simulink model "Temperature_Controller"  (R2024b)
settings: Solver=VariableStepAuto  StartTime=0.0  StopTime=inf  RelTol=1e-3
libraries: arduinolib x3, simulink x1
settings Model: Creator=John Coetzee  LastModifiedBy=John Coetzee

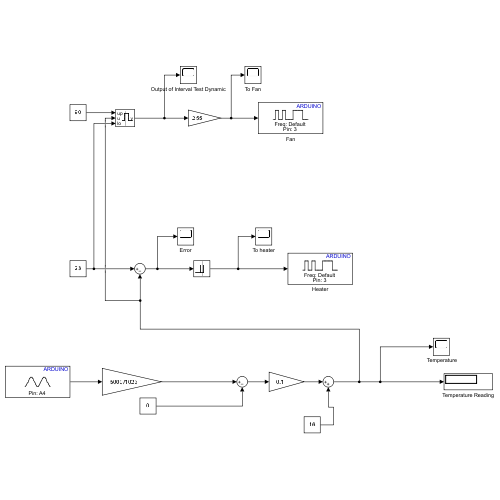
[thumbnail: Simulink's stored preview of the top-level diagram]
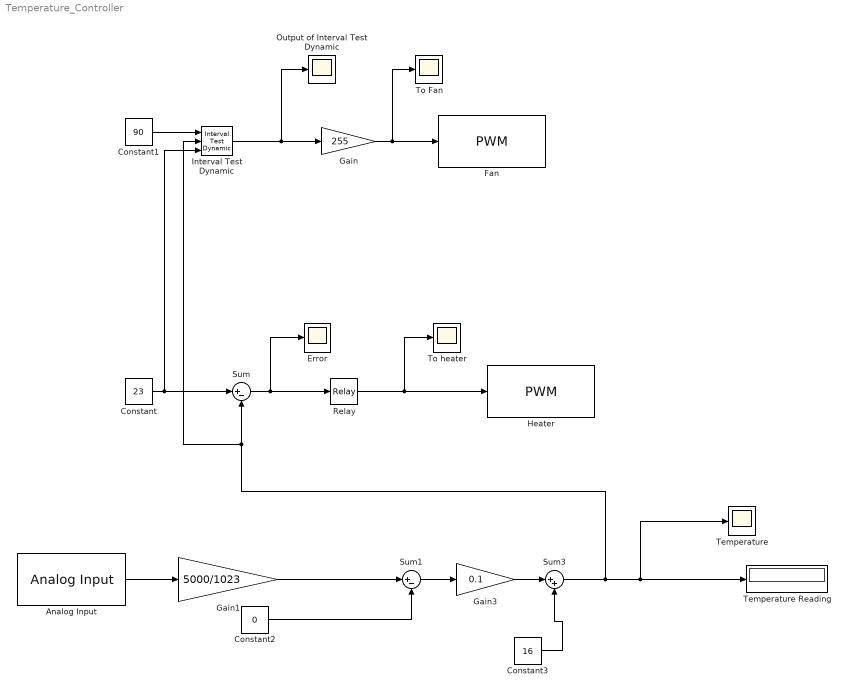
== system Temperature_Controller ==
  " Temperature" : Scope
  Analog Input : arduinolib/Analog Input  pinNumber=4  ReadResultsOnly=off  ConversionTriggerSource=Software  ExternalTriggerType=uint32( 0 )  OutputDataType=uint16  EnableConversionCompleteNotify=off  EnableOuputStatus=off  SampleTime=-1  blockPlatform=arduino
      settings: SourceProductName=Common
  Constant : Constant  Value=23
  Constant1 : Constant  Value=90
  Constant2 : Constant  Value=0
  Constant3 : Constant  Value=16
  Error : Scope
  Fan : arduinolib/PWM  pinNumber=3  frequencyType=Default  desiredFrequency=490.2  achievableFrequency=490.2
      settings: SourceProductName=Common
  Gain : Gain  Gain=255
  Gain1 : Gain  Gain=5000/1023
  Gain3 : Gain  Gain=0.1
  Heater : arduinolib/PWM  pinNumber=3  frequencyType=Default  desiredFrequency=490.2  achievableFrequency=490.2
      settings: SourceProductName=Common
  Interval Test Dynamic : simulink/Logic and Bit Operations/Interval Test Dynamic  IntervalClosedRight=on  IntervalClosedLeft=on  OutDataTypeStr=boolean
  Output of Interval Test Dynamic : Scope
  Relay : Relay  OnSwitchValue=0.1  OffSwitchValue=0.0001  OnOutputValue=255
  Sum : Sum  Inputs=|+-
  Sum1 : Sum  Inputs=|+-
  Sum3 : Sum  Inputs=|++
  Temperature Reading : Display
  To Fan : Scope
  To heater : Scope
  wires:
  Constant/1 -> Interval Test Dynamic/3, Sum/1
  Sum/1 -> Error/1, Relay/1
  Constant1/1 -> Interval Test Dynamic/1
  Interval Test Dynamic/1 -> Output of Interval Test Dynamic/1, Gain/1
  Analog Input/1 -> Gain1/1
  Constant2/1 -> Sum1/2
  Gain1/1 -> Sum1/1
  Relay/1 -> To heater/1, Heater/1
  Gain/1 -> Fan/1, To Fan/1
  Constant3/1 -> Sum3/2
  Sum3/1 -> " Temperature"/1, Temperature Reading/1, Interval Test Dynamic/2, Sum/2
  Sum1/1 -> Gain3/1
  Gain3/1 -> Sum3/1
